simulink model "ThesisComparison"  (R2017a)
settings: Solver=VariableStepAuto  StartTime=0.0  StopTime=10.0  RelTol=1e-3
undefined symbols (not defined in the file): DiscIntNeverNeededParam
libraries: dspmlti4 x2, dsparch4 x1
settings Model: Creator=bhannigan  LastModifiedBy=bhannigan

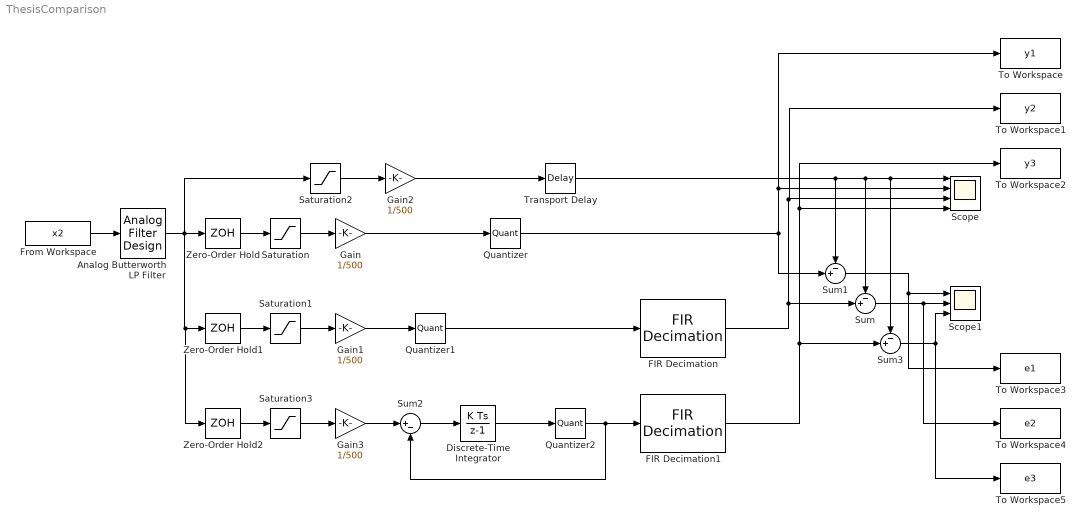
== system ThesisComparison ==
  Analog Butterworth LP Filter : dsparch4/Analog Filter Design  method=Butterworth  filttype=Lowpass  N=6  Wlo=2*pi*50  Whi=80  Rp=2  Rs=40
  Discrete-Time Integrator : DiscreteIntegrator  gainval=1000  InitialConditionSetting=State (most efficient)  SampleTime=1/1000  ICPrevOutput=DiscIntNeverNeededParam  ICPrevScaledInput=DiscIntNeverNeededParam
  FIR Decimation : dspmlti4/FIR Decimation  FilterSource=Dialog parameters  h=fir1(31,0.25)  D=10  filtStruct=Direct form  FilterObject=FDECIM  framing=Enforce single-rate processing  inputOffset=0  outputBufInitCond=0  roundingMode=Floor  overflowMode=off  firstCoeffDataTypeStr=Inherit: Same word length as input  firstCoeffMin=[]  firstCoeffMax=[]  firstCoeffLastDataTypeStr=Inherit: Same word length as input  outputDataTypeStr=Inherit: Same as accumulator  outputMin=[]  outputMax=[]  outputLastDataTypeStr=Inherit: Same as accumulator
  FIR Decimation1 : dspmlti4/FIR Decimation  FilterSource=Dialog parameters  h=fir1(31,0.25)  D=10  filtStruct=Direct form  FilterObject=FDECIM  framing=Enforce single-rate processing  inputOffset=0  outputBufInitCond=0  roundingMode=Floor  overflowMode=off  firstCoeffDataTypeStr=Inherit: Same word length as input  firstCoeffMin=[]  firstCoeffMax=[]  firstCoeffLastDataTypeStr=Inherit: Same word length as input  outputDataTypeStr=Inherit: Same as accumulator  outputMin=[]  outputMax=[]  outputLastDataTypeStr=Inherit: Same as accumulator
  From Workspace : FromWorkspace  VariableName=x2  SampleTime=1/1000
  Gain{,1..3} (4 alike) : Gain  Gain=1/500
  Quantizer : Quantizer  QuantizationInterval=0.0625
  Quantizer1 : Quantizer  QuantizationInterval=0.0625
  Quantizer2 : Quantizer  QuantizationInterval=0.0625
  Saturation{,1..3} (4 alike) : Saturate  UpperLimit=500  LowerLimit=-500
  Scope : Scope  NumInputPorts=4
  Scope1 : Scope  NumInputPorts=3
  Sum : Sum  Inputs=-+|
  Sum1 : Sum  Inputs=-+|
  Sum2 : Sum  Inputs=|+-
  Sum3 : Sum  Inputs=-+|
  To Workspace : ToWorkspace  VariableName=y1  SaveFormat=Timeseries  SampleTime=-1
  To Workspace1 : ToWorkspace  VariableName=y2  SaveFormat=Timeseries  SampleTime=-1
  To Workspace2 : ToWorkspace  VariableName=y3  SaveFormat=Timeseries  SampleTime=-1
  To Workspace3 : ToWorkspace  VariableName=e1  SaveFormat=Timeseries  SampleTime=-1
  To Workspace4 : ToWorkspace  VariableName=e2  SaveFormat=Timeseries  SampleTime=-1
  To Workspace5 : ToWorkspace  VariableName=e3  SaveFormat=Timeseries  SampleTime=-1
  Transport Delay : TransportDelay  DelayTime=16/1000
  Zero-Order Hold : ZeroOrderHold  SampleTime=1/100
  Zero-Order Hold1 : ZeroOrderHold  SampleTime=1/1000
  Zero-Order Hold2 : ZeroOrderHold  SampleTime=1/1000
  wires:
  From Workspace/1 -> Analog Butterworth LP Filter/1
  Analog Butterworth LP Filter/1 -> Saturation2/1, Zero-Order Hold2/1, Zero-Order Hold1/1, Zero-Order Hold/1
  Saturation/1 -> Gain/1
  Gain/1 -> Quantizer/1
  Zero-Order Hold/1 -> Saturation/1
  Saturation1/1 -> Gain1/1
  Zero-Order Hold1/1 -> Saturation1/1
  Gain1/1 -> Quantizer1/1
  Quantizer1/1 -> FIR Decimation/1
  Quantizer/1 -> To Workspace/1, Scope/2, Sum1/2
  Gain2/1 -> Transport Delay/1
  Saturation2/1 -> Gain2/1
  FIR Decimation/1 -> To Workspace1/1, Scope/3, Sum/2
  Transport Delay/1 -> Sum1/1, Sum/1, Scope/1, Sum3/1
  Sum1/1 -> To Workspace3/1, Scope1/1
  Saturation3/1 -> Gain3/1
  Zero-Order Hold2/1 -> Saturation3/1
  Gain3/1 -> Sum2/1
  Sum2/1 -> Discrete-Time Integrator/1
  Discrete-Time Integrator/1 -> Quantizer2/1
  Quantizer2/1 -> FIR Decimation1/1, Sum2/2
  FIR Decimation1/1 -> Scope/4, To Workspace2/1, Sum3/2
  Sum3/1 -> To Workspace5/1, Scope1/3
  Sum/1 -> To Workspace4/1, Scope1/2
